simulink model "pendulum"  (R2022b)
settings: Solver=VariableStepAuto  StartTime=0.0  StopTime=stoptime  RelTol=1e-3
values from neighbouring files (symbols this model uses):
  d_theta0 = 0    [pendulum_main.m]
  theta0 = 1.57    [pendulum_main.m]
settings Model: Creator=a1pab  LastModifiedBy=a1pab

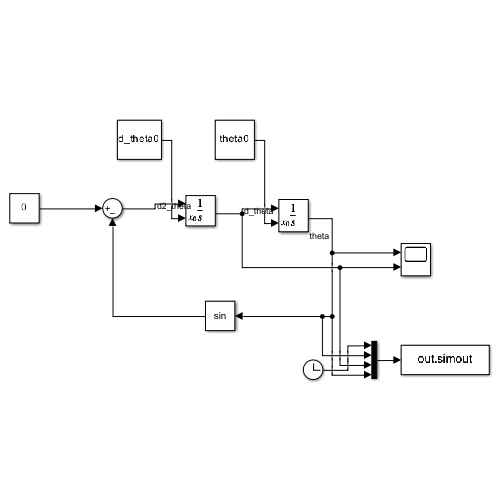
[thumbnail: Simulink's stored preview of the top-level diagram]
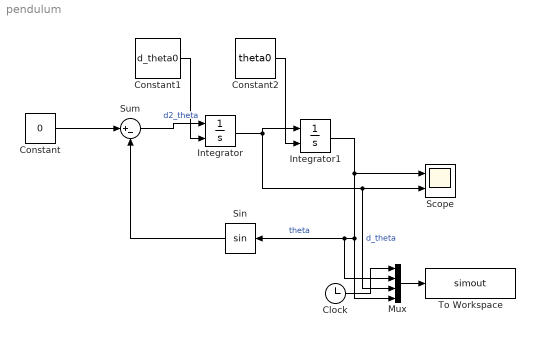
== system pendulum ==
  Clock : Clock
  Constant : Constant  Value=0
  Constant1 : Constant  Value=d_theta0
  Constant2 : Constant  Value=theta0
  Integrator : Integrator  InitialConditionSource=external
  Integrator1 : Integrator  InitialConditionSource=external  InitialCondition=theta0
  Mux : Mux
  Scope : Scope  NumInputPorts=2
  Sin : Trigonometry
  Sum : Sum  Inputs=|+-
  To Workspace : ToWorkspace  VariableName=simout  SampleTime=-1
  wires:
  Constant/1 -> Sum/1
  Sin/1 -> Sum/2
  Sum/1 -> Integrator/1  "d2_theta"
  Integrator/1 -> Integrator1/1, Scope/2, Mux/3  "d_theta"
  Integrator1/1 -> Mux/4, Mux/2, Sin/1, Scope/1  "theta"
  Mux/1 -> To Workspace/1
  Clock/1 -> Mux/1
  Constant1/1 -> Integrator/2
  Constant2/1 -> Integrator1/2
